simulink model "GetSineWaveFcn"  (R2021a)
settings: Solver=FixedStepDiscrete  StartTime=0.0  StopTime=10.0  FixedStep=0.1  RelTol=1e-3  EnableMultiTasking=on
settings Model: Creator=kylec  LastModifiedBy=kylec
settings SolverCC: AlgebraicLoopSolver=TrustRegion  AutoInsertRateTranBlk=on
settings DataIOCC: LimitDataPoints=on
settings OptimizationCC: LifeSpan=inf
settings DebuggingCC: AllowSymbolicDim=off  SFUnexpectedBacktrackingDiag=warning  SFNoUnconditionalDefaultTransitionDiag=warning  SFExecutionAtInitializationDiag=none  ArithmeticOperatorsInVariantConditions=warning
settings SFSimCC: SimUseLocalCustomCode=off  CustomCodeUndefinedFunction=UseInterfaceOnly
settings RTWCC: RTWUseLocalCustomCode=off
settings CodeAppCC: StateflowObjectComments=on
settings GRTTargetCC: TargetLangStandard=C89/C90 (ANSI)
settings ConfigComp: CovMetricSettings=dw  CovSaveCumulativeToWorkspaceVar=on  CovSaveSingleToWorkspaceVar=on  CovExternalEMLEnable=off

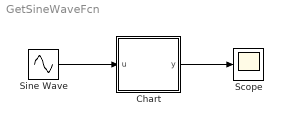
== system GetSineWaveFcn ==
  Chart : Stateflow chart  TreatAsAtomicUnit=on
  Scope : Scope
  Sine Wave : Sin  SampleTime=0
  wires:
  Sine Wave/1 -> Chart/1(u)
  Chart/1(y) -> Scope/1

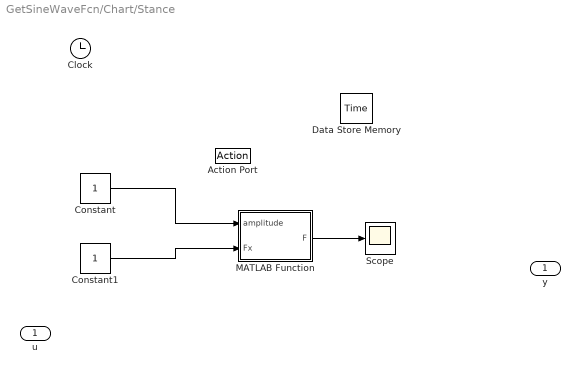
== system GetSineWaveFcn/Chart/Stance ==
  u : Inport
  Action Port : ActionPort
      settings: CopyFcn=Stateflow.SLINSF.SimulinkMan.removeBlockPreDeleteFcn  PreDeleteFcn=Stateflow.SLINSF.SimulinkMan.unsafePredeleteFcn
  Clock : Clock
  Constant : Constant
  Constant1 : Constant
  Data Store Memory : DataStoreMemory  DataStoreName=Time  ReadBeforeWriteMsg=warning  WriteAfterWriteMsg=warning  WriteAfterReadMsg=warning  ShowAdditionalParam=off
  MATLAB Function : MATLAB Function  TreatAsAtomicUnit=on
  Scope : Scope
  y : Outport
  wires:
  Constant/1 -> MATLAB Function/1(amplitude)
  Constant1/1 -> MATLAB Function/2(Fx)
  MATLAB Function/1(F) -> Scope/1

== matlab function GetSineWaveFcn/Chart/Stance/MATLAB Function ==
  data: amplitude input; F output; Fx input

function F = grf(amplitude, Fx)
t = 1:0.05:4;
f = 0.5;
y=amplitude * sin(2*pi*f*t);% Generate Sine Wave  
y(y<0) = 0;                       % Rectified Sine Wave
%plot(t,y);
F = y;
 
end

== stateflow chart GetSineWaveFcn/Chart ==
  state Flight %State Name
    entry: y = -1; % entry action
    % during:
  state Stance
  (default) -> Flight %State Name
  Flight %State Name -> Stance : [ydot < 0 && yfoot <= 0]% [transition condition]{action}
  Stance -> Flight %State Name : [GRFy == 0 && ydot > 0]
  data: sf_internal_action_state_placeholder_data local double size=1 =0; u input; y output
